simulink model "copper_solvent_extraction_model_simulink"  (R2021a)
settings: Solver=ode14x  StartTime=0.0  StopTime=simulation_time  FixedStep=step_time  RelTol=1e-3
undefined symbols (not defined in the file): C1_aq_ss, C1_el_ss, C1_org_ss, C2_aq_ss, C2_org_ss, C3_aq_ss, C3_org_ss, C4_org_ss, C_aq_max, C_org_max, cLE_ss, cPLS_ss, EXTERNAL_VARIABLES_STEADY_STATE, fLE_max, fLO_max, fPLSP_ss, fPLSS_ss, I_FB1, I_FB2, K_eq_ext, K_eq_str, K_ff_FF1, K_ff_FF2, K_ff_FF3, K_ff_FF4, K_mass_1, K_mass_2, K_mass_3, K_mass_4, Kb_FB1, Kb_FB2, Kc_FB1, Kc_FB2, seed_c_BO, seed_c_LE, seed_c_LO, seed_c_PLS, seed_c_RaffP, seed_c_RaffS, seed_c_RE, seed_f_LE, seed_f_LO, seed_f_PLSP, seed_f_PLSS, sigma_c_BO, sigma_c_LE, sigma_c_LO, sigma_c_PLS, sigma_c_RaffP, sigma_c_RaffS, sigma_c_RE, sigma_f_LE, sigma_f_LO, sigma_f_PLSP, sigma_f_PLSS, step_time, t1, t2, t3, t4 ... (+22)
libraries: slpidlib x2
(part 2 of 2)

== system copper_solvent_extraction_model_simulink/Valve LE ==
  vLE_control_saturated(t) : Inport
  Memory : Memory  InitialCondition=vLE_ss
  Simulation time : Clock
  Valve LE flow model : Subsystem
      mask Display: image('C:\Users\piete\Desktop\Programming\Engineering\Process-State-Identification\assets\simulink\valves\valve_LE_flow_model.png'); % Use "Edit Image" on toolstrip to change.
  Valve LE valve model : Subsystem
      settings: PortSchema="{\"entries\":[{\"content\":{\"sides\":[{\"content\":{\"connectorIds\":[\"In1\"]},\"type\":\"ConnectorPlacement.EquallySpacedRectSide\",\"uuid\":\"2e9f031d-8496-4052-a2e0-829d2345863a\"},{\"content\":{\"connectorIds\":[\"Out1\"],\"side\":\"RIGHT\"},\"type\":\"ConnectorPlacement.EquallySpacedRectSide\",\"uuid\":\"38b5eb17-cc51-4fa3-9394-ca0ed547bb78\"},{\"content\":{\"connectorIds\":[\"In2\",\"In3\"],\"side\":\"TOP\"},\"type\":\"ConnectorPlacement.EquallySpacedRectSide\",\"uuid\":\"bfeaaf73-7bd9-4ee3-b412-f379f1bcce90\"}]},\"type\":\"ConnectorPlacement.EquallySpacedConnector\",\"uuid\":\"a9e57682-026b-43fa-bec2-e5bd18169bdc\"}],\"packageUris\":[\"http://schema.mathworks.com/mf0/Connector/R2020b\"],\"version\":\"1.0\"}"
      mask Display: image('C:\Users\piete\Desktop\Programming\Engineering\Process-State-Identification\assets\simulink\valves\valve_LE_valve_model.png'); % Use "Edit Image" on toolstrip to change.
  Variant Subsystem : Subsystem  Variant=on
      mask Display: image('.\assets\simulink\valves\valve_LE_state.png'); % Use "Edit Image" on toolstrip to change.
  fLE(t) : Outport
  wires:
  Valve LE flow model/1(fLE(t)) -> fLE(t)/1  "fLE(t)"
  Variant Subsystem/1(valve_LE_state) -> Valve LE valve model/2(valve_LE_state)  "valve_LE_state(t)"
  Simulation time/1 -> Variant Subsystem/1(simulation_time)  "simulation_time"
  Variant Subsystem/2(v_LE_is_not_stuck) -> Valve LE valve model/3(v_LE_is_not_stuck(t))  "v_LE_is_not_stuck(t)"
  Memory/1 -> Variant Subsystem/2(v_LE_valve_previous)  "v_LE_valve_previous(t)"
  Valve LE valve model/1(v_LE_valve(t)) -> Memory/1, Valve LE flow model/1(vLE_valve(t))  "v_LE_valve(t)"
  vLE_control_saturated(t)/1 -> Valve LE valve model/1(v_LE_control(t))  "vLE_control_saturated(t)"

== system copper_solvent_extraction_model_simulink/Valve LO ==
  vLO_control_saturated(t) : Inport
  Memory : Memory  InitialCondition=vLO_ss
  Simulation time : Clock
  Valve LO flow model : Subsystem
      mask Display: image('.\assets\simulink\valves\valve_LO_flow_model.png'); % Use "Edit Image" on toolstrip to change.
  Valve LO valve model : Subsystem
      settings: PortSchema="{\"entries\":[{\"content\":{\"sides\":[{\"content\":{\"connectorIds\":[\"In1\"]},\"type\":\"ConnectorPlacement.EquallySpacedRectSide\",\"uuid\":\"2e9f031d-8496-4052-a2e0-829d2345863a\"},{\"content\":{\"connectorIds\":[\"Out1\"],\"side\":\"RIGHT\"},\"type\":\"ConnectorPlacement.EquallySpacedRectSide\",\"uuid\":\"38b5eb17-cc51-4fa3-9394-ca0ed547bb78\"},{\"content\":{\"connectorIds\":[\"In2\",\"In3\"],\"side\":\"TOP\"},\"type\":\"ConnectorPlacement.EquallySpacedRectSide\",\"uuid\":\"bfeaaf73-7bd9-4ee3-b412-f379f1bcce90\"}]},\"type\":\"ConnectorPlacement.EquallySpacedConnector\",\"uuid\":\"a9e57682-026b-43fa-bec2-e5bd18169bdc\"}],\"packageUris\":[\"http://schema.mathworks.com/mf0/Connector/R2020b\"],\"version\":\"1.0\"}"
      mask Display: image('.\assets\simulink\valves\valve_LO_valve_model.png'); % Use "Edit Image" on toolstrip to change.
  Variant Subsystem : Subsystem  Variant=on
      mask Display: image('.\assets\simulink\valves\valve_LO_state.png'); % Use "Edit Image" on toolstrip to change.
  f_LO(t) : Outport
  wires:
  Valve LO flow model/1(fLO(t)) -> f_LO(t)/1  "f_LO(t)"
  vLO_control_saturated(t)/1 -> Valve LO valve model/1(v_LO_control(t))  "vLO_control_saturated(t)"
  Valve LO valve model/1(v_LO_valve(t)) -> Memory/1, Valve LO flow model/1(vLO_valve(t))  "v_LO_valve(t)"
  Variant Subsystem/1(valve_LO_state) -> Valve LO valve model/2(valve_LO_state)  "valve_LO_state(t)"
  Simulation time/1 -> Variant Subsystem/1(simulation_time)  "simulation_time"
  Variant Subsystem/2(v_LO_is_not_stuck) -> Valve LO valve model/3(v_LO_is_not_stuck(t))  "v_LO_is_not_stuck(t)"
  Memory/1 -> Variant Subsystem/2(v_LO_valve_previous)  "v_LO_valve_previous(t)"

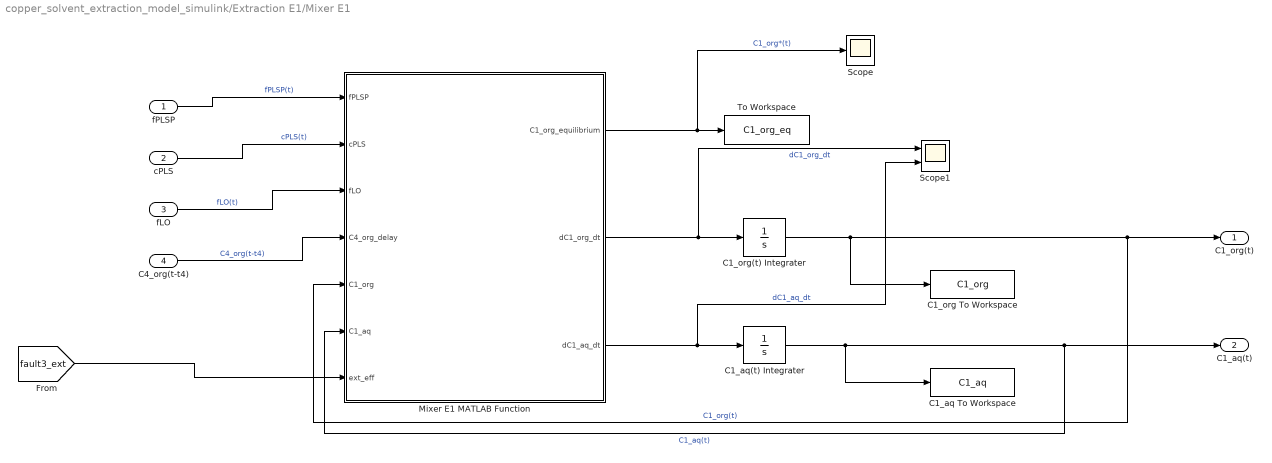
== system copper_solvent_extraction_model_simulink/Extraction E1/Mixer E1 ==
  fPLSP : Inport
  cPLS : Inport  Port=2
  fLO : Inport  Port=3
  C4_org(t-t4) : Inport  Port=4
  C1_aq To Workspace : ToWorkspace  VariableName=C1_aq  SaveFormat=Timeseries  SampleTime=-1
  C1_aq(t) Integrater : Integrator  InitialCondition=C1_aq_ss
  C1_org To Workspace : ToWorkspace  VariableName=C1_org  SaveFormat=Timeseries  SampleTime=-1
  C1_org(t) Integrater : Integrator  InitialCondition=C1_org_ss
  Mixer E1 MATLAB Function : MATLAB Function  TreatAsAtomicUnit=on
  Scope : Scope
  Scope1 : Scope  NumInputPorts=2
  To Workspace : ToWorkspace  VariableName=C1_org_eq  SaveFormat=Timeseries  SampleTime=-1
  C1_org(t) : Outport
  C1_aq(t) : Outport  Port=2
  wires:
  C1_org(t) Integrater/1 -> C1_org(t)/1, Mixer E1 MATLAB Function/5(C1_org), C1_org To Workspace/1  "C1_org(t)"
  Mixer E1 MATLAB Function/2(dC1_org_dt) -> Scope1/1, C1_org(t) Integrater/1  "dC1_org_dt"
  C1_aq(t) Integrater/1 -> C1_aq(t)/1, Mixer E1 MATLAB Function/6(C1_aq), C1_aq To Workspace/1  "C1_aq(t)"
  Mixer E1 MATLAB Function/1(C1_org_equilibrium) -> Scope/1, To Workspace/1  "C1_org*(t)"
  Mixer E1 MATLAB Function/3(dC1_aq_dt) -> Scope1/2, C1_aq(t) Integrater/1  "dC1_aq_dt"
  C4_org(t-t4)/1 -> Mixer E1 MATLAB Function/4(C4_org_delay)  "C4_org(t-t4)"
  fLO/1 -> Mixer E1 MATLAB Function/3(fLO)  "fLO(t)"
  cPLS/1 -> Mixer E1 MATLAB Function/2(cPLS)  "cPLS(t)"
  fPLSP/1 -> Mixer E1 MATLAB Function/1(fPLSP)  "fPLSP(t)"
  [fault3_ext] -> Mixer E1 MATLAB Function/7(ext_eff)

== system copper_solvent_extraction_model_simulink/Extraction E1/Sensor c_RaffP ==
  c_RaffP(t) : Inport
  Random Number : RandomNumber  Variance=sigma_c_RaffP^2  Seed=seed_c_RaffP  SampleTime=step_time
  Saturation : Saturate  UpperLimit=inf  LowerLimit=0
  Sum : Sum  Inputs=++|
  To Workspace : ToWorkspace  VariableName=c_RaffP_measured  SaveFormat=Timeseries  SampleTime=-1
  wires:
  c_RaffP(t)/1 -> Sum/2  "c_RaffP(t)"
  Random Number/1 -> Sum/1  "Sensor c_RaffP Noise"
  Sum/1 -> Saturation/1  "c_RaffP_measured(t)"
  Saturation/1 -> To Workspace/1  "c_RaffP_measured_bounded(t)"

== system copper_solvent_extraction_model_simulink/Extraction E1/Settler E1 ==
  C1_org(t) : Inport
  C1_aq(t) : Inport  Port=2
  C1_aq_delay To Workspace : ToWorkspace  VariableName=C1_aq_delay  SaveFormat=Timeseries  SampleTime=-1
  C1_org_delay To Workspace : ToWorkspace  VariableName=C1_org_delay  SaveFormat=Timeseries  SampleTime=-1
  E1 Aqueous Settler : TransportDelay  DelayTime=t1  InitialOutput=C1_aq_ss
  E1 Organic Settler : TransportDelay  DelayTime=t1  InitialOutput=C1_org_ss
  C1_org(t-t1) : Outport
  C1_aq(t-t1) : Outport  Port=2
  wires:
  C1_org(t)/1 -> E1 Organic Settler/1  "C1_org(t)"
  E1 Organic Settler/1 -> C1_org_delay To Workspace/1, C1_org(t-t1)/1  "C1_org(t-t1)"
  E1 Aqueous Settler/1 -> C1_aq(t-t1)/1, C1_aq_delay To Workspace/1  "C1_aq(t-t1)"
  C1_aq(t)/1 -> E1 Aqueous Settler/1  "C1_aq(t)"

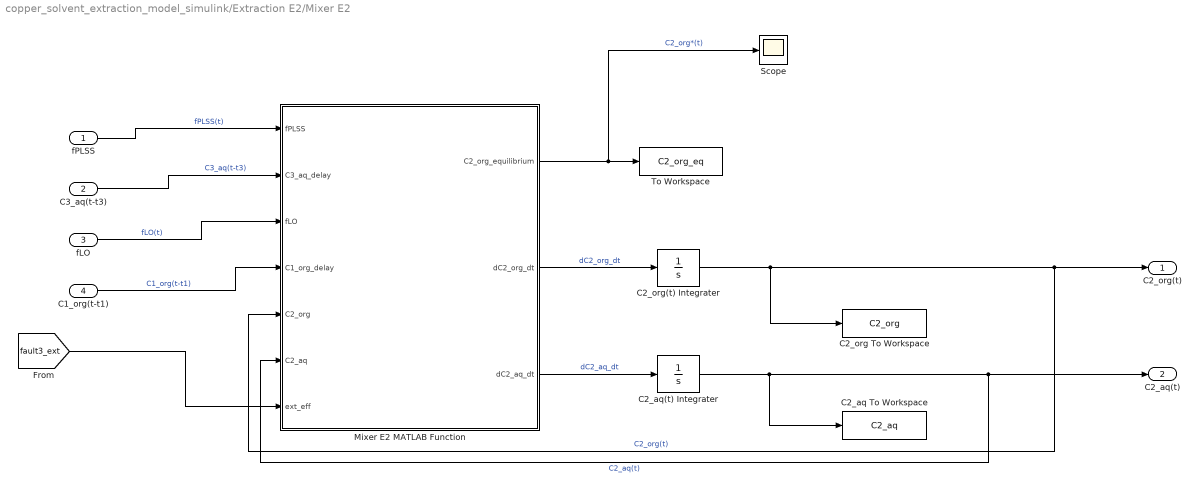
== system copper_solvent_extraction_model_simulink/Extraction E2/Mixer E2 ==
  fPLSS : Inport
  C3_aq(t-t3) : Inport  Port=2
  fLO : Inport  Port=3
  C1_org(t-t1) : Inport  Port=4
  C2_aq To Workspace : ToWorkspace  VariableName=C2_aq  SaveFormat=Timeseries  SampleTime=-1
  C2_aq(t) Integrater : Integrator  InitialCondition=C2_aq_ss
  C2_org To Workspace : ToWorkspace  VariableName=C2_org  SaveFormat=Timeseries  SampleTime=-1
  C2_org(t) Integrater : Integrator  InitialCondition=C2_org_ss
  Mixer E2 MATLAB Function : MATLAB Function  TreatAsAtomicUnit=on
  Scope : Scope
  To Workspace : ToWorkspace  VariableName=C2_org_eq  SaveFormat=Timeseries  SampleTime=-1
  C2_org(t) : Outport
  C2_aq(t) : Outport  Port=2
  wires:
  C2_aq(t) Integrater/1 -> Mixer E2 MATLAB Function/6(C2_aq), C2_aq(t)/1, C2_aq To Workspace/1  "C2_aq(t)"
  C2_org(t) Integrater/1 -> C2_org(t)/1, Mixer E2 MATLAB Function/5(C2_org), C2_org To Workspace/1  "C2_org(t)"
  fLO/1 -> Mixer E2 MATLAB Function/3(fLO)  "fLO(t)"
  Mixer E2 MATLAB Function/3(dC2_aq_dt) -> C2_aq(t) Integrater/1  "dC2_aq_dt"
  Mixer E2 MATLAB Function/1(C2_org_equilibrium) -> Scope/1, To Workspace/1  "C2_org*(t)"
  Mixer E2 MATLAB Function/2(dC2_org_dt) -> C2_org(t) Integrater/1  "dC2_org_dt"
  fPLSS/1 -> Mixer E2 MATLAB Function/1(fPLSS)  "fPLSS(t)"
  C3_aq(t-t3)/1 -> Mixer E2 MATLAB Function/2(C3_aq_delay)  "C3_aq(t-t3)"
  C1_org(t-t1)/1 -> Mixer E2 MATLAB Function/4(C1_org_delay)  "C1_org(t-t1)"
  [fault3_ext] -> Mixer E2 MATLAB Function/7(ext_eff)

== system copper_solvent_extraction_model_simulink/Extraction E2/Sensor c_RaffS ==
  c_RaffS(t) : Inport
  Random Number : RandomNumber  Variance=sigma_c_RaffS^2  Seed=seed_c_RaffS  SampleTime=step_time
  Saturation : Saturate  UpperLimit=inf  LowerLimit=0
  Sum : Sum  Inputs=++|
  To Workspace : ToWorkspace  VariableName=c_RaffS_measured  SaveFormat=Timeseries  SampleTime=-1
  wires:
  c_RaffS(t)/1 -> Sum/2  "c_RaffS(t)"
  Random Number/1 -> Sum/1  "Sensor c_RaffS Noise"
  Sum/1 -> Saturation/1  "c_RaffS_measured(t)"
  Saturation/1 -> To Workspace/1  "c_RaffS_measured_bounded(t)"

== system copper_solvent_extraction_model_simulink/Extraction E2/Settler E2 ==
  C2_org(t) : Inport
  C2_aq(t) : Inport  Port=2
  C2_aq_delay To Workspace : ToWorkspace  VariableName=C2_aq_delay  SaveFormat=Timeseries  SampleTime=-1
  C2_org_delay To Workspace : ToWorkspace  VariableName=C2_org_delay  SaveFormat=Timeseries  SampleTime=-1
  E2 Aqueous Settler : TransportDelay  DelayTime=t2  InitialOutput=C2_aq_ss
  E2 Organic Settler : TransportDelay  DelayTime=t2  InitialOutput=C2_org_ss
  C2_org(t-t2) : Outport
  C2_aq(t-t2) : Outport  Port=2
  wires:
  E2 Aqueous Settler/1 -> C2_aq(t-t2)/1, C2_aq_delay To Workspace/1  "C2_aq(t-t2)"
  C2_aq(t)/1 -> E2 Aqueous Settler/1  "C2_aq(t)"
  C2_org(t)/1 -> E2 Organic Settler/1  "C2_org(t)"
  E2 Organic Settler/1 -> C2_org_delay To Workspace/1, C2_org(t-t2)/1  "C2_org(t-t2)"

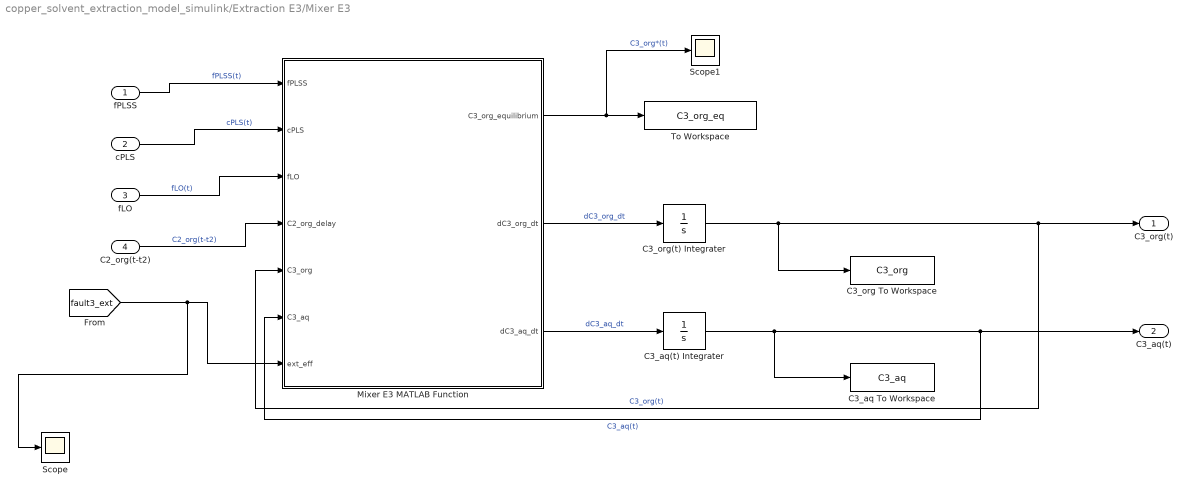
== system copper_solvent_extraction_model_simulink/Extraction E3/Mixer E3 ==
  fPLSS : Inport
  cPLS : Inport  Port=2
  fLO : Inport  Port=3
  C2_org(t-t2) : Inport  Port=4
  C3_aq To Workspace : ToWorkspace  VariableName=C3_aq  SaveFormat=Timeseries  SampleTime=-1
  C3_aq(t) Integrater : Integrator  InitialCondition=C3_aq_ss
  C3_org To Workspace : ToWorkspace  VariableName=C3_org  SaveFormat=Timeseries  SampleTime=-1
  C3_org(t) Integrater : Integrator  InitialCondition=C3_org_ss
  Mixer E3 MATLAB Function : MATLAB Function  TreatAsAtomicUnit=on
  Scope : Scope
  Scope1 : Scope
  To Workspace : ToWorkspace  VariableName=C3_org_eq  SaveFormat=Timeseries  SampleTime=-1
  C3_org(t) : Outport
  C3_aq(t) : Outport  Port=2
  wires:
  C3_aq(t) Integrater/1 -> Mixer E3 MATLAB Function/6(C3_aq), C3_aq(t)/1, C3_aq To Workspace/1  "C3_aq(t)"
  C3_org(t) Integrater/1 -> Mixer E3 MATLAB Function/5(C3_org), C3_org(t)/1, C3_org To Workspace/1  "C3_org(t)"
  Mixer E3 MATLAB Function/2(dC3_org_dt) -> C3_org(t) Integrater/1  "dC3_org_dt"
  C2_org(t-t2)/1 -> Mixer E3 MATLAB Function/4(C2_org_delay)  "C2_org(t-t2)"
  Mixer E3 MATLAB Function/3(dC3_aq_dt) -> C3_aq(t) Integrater/1  "dC3_aq_dt"
  cPLS/1 -> Mixer E3 MATLAB Function/2(cPLS)  "cPLS(t)"
  fLO/1 -> Mixer E3 MATLAB Function/3(fLO)  "fLO(t)"
  fPLSS/1 -> Mixer E3 MATLAB Function/1(fPLSS)  "fPLSS(t)"
  Mixer E3 MATLAB Function/1(C3_org_equilibrium) -> Scope1/1, To Workspace/1  "C3_org*(t)"
  [fault3_ext] -> Scope/1, Mixer E3 MATLAB Function/7(ext_eff)

== system copper_solvent_extraction_model_simulink/Extraction E3/Settler E3 ==
  C3_org(t) : Inport
  C3_aq(t) : Inport  Port=2
  C3_aq_delay To Workspace : ToWorkspace  VariableName=C3_aq_delay  SaveFormat=Timeseries  SampleTime=-1
  C3_org_delay To Workspace : ToWorkspace  VariableName=C3_org_delay  SaveFormat=Timeseries  SampleTime=-1
  E3 Aqueous Settler : TransportDelay  DelayTime=t3  InitialOutput=C3_aq_ss
  E3 Organic Settler : TransportDelay  DelayTime=t3  InitialOutput=C3_org_ss
  C3_org(t-t3) : Outport
  C3_aq(t-t3) : Outport  Port=2
  wires:
  C3_aq(t)/1 -> E3 Aqueous Settler/1  "C3_aq(t)"
  E3 Aqueous Settler/1 -> C3_aq(t-t3)/1, C3_aq_delay To Workspace/1  "C3_aq(t-t3)"
  E3 Organic Settler/1 -> C3_org(t-t3)/1, C3_org_delay To Workspace/1  "C3_org(t-t3)"
  C3_org(t)/1 -> E3 Organic Settler/1  "C3_org(t)"

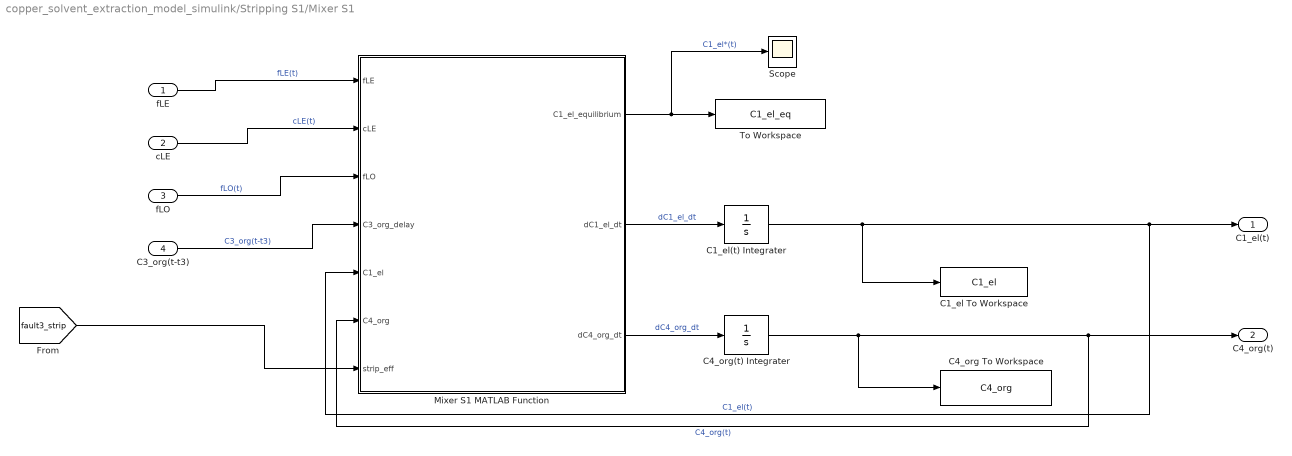
== system copper_solvent_extraction_model_simulink/Stripping S1/Mixer S1 ==
  fLE : Inport
  cLE : Inport  Port=2
  fLO : Inport  Port=3
  C3_org(t-t3) : Inport  Port=4
  C1_el To Workspace : ToWorkspace  VariableName=C1_el  SaveFormat=Timeseries  SampleTime=-1
  C1_el(t) Integrater : Integrator  InitialCondition=C1_el_ss
  C4_org To Workspace : ToWorkspace  VariableName=C4_org  SaveFormat=Timeseries  SampleTime=-1
  C4_org(t) Integrater : Integrator  InitialCondition=C4_org_ss
  Mixer S1 MATLAB Function : MATLAB Function  TreatAsAtomicUnit=on
  Scope : Scope
  To Workspace : ToWorkspace  VariableName=C1_el_eq  SaveFormat=Timeseries  SampleTime=-1
  C1_el(t) : Outport
  C4_org(t) : Outport  Port=2
  wires:
  C3_org(t-t3)/1 -> Mixer S1 MATLAB Function/4(C3_org_delay)  "C3_org(t-t3)"
  Mixer S1 MATLAB Function/2(dC1_el_dt) -> C1_el(t) Integrater/1  "dC1_el_dt"
  C4_org(t) Integrater/1 -> Mixer S1 MATLAB Function/6(C4_org), C4_org(t)/1, C4_org To Workspace/1  "C4_org(t)"
  C1_el(t) Integrater/1 -> Mixer S1 MATLAB Function/5(C1_el), C1_el(t)/1, C1_el To Workspace/1  "C1_el(t)"
  cLE/1 -> Mixer S1 MATLAB Function/2(cLE)  "cLE(t)"
  Mixer S1 MATLAB Function/1(C1_el_equilibrium) -> Scope/1, To Workspace/1  "C1_el*(t)"
  Mixer S1 MATLAB Function/3(dC4_org_dt) -> C4_org(t) Integrater/1  "dC4_org_dt"
  fLO/1 -> Mixer S1 MATLAB Function/3(fLO)  "fLO(t)"
  fLE/1 -> Mixer S1 MATLAB Function/1(fLE)  "fLE(t)"
  [fault3_strip] -> Mixer S1 MATLAB Function/7(strip_eff)

== system copper_solvent_extraction_model_simulink/Stripping S1/Settler S1 ==
  C1_el(t) : Inport
  C4_org(t) : Inport  Port=2
  C1_el_delay To Workspace : ToWorkspace  VariableName=C1_el_delay  SaveFormat=Timeseries  SampleTime=-1
  C4_org_delay To Workspace : ToWorkspace  VariableName=C4_org_delay  SaveFormat=Timeseries  SampleTime=-1
  S1 Electrolyte Settler : TransportDelay  DelayTime=t4  InitialOutput=C1_el_ss
  S1 Organic Settler : TransportDelay  DelayTime=t4  InitialOutput=C4_org_ss
  C1_el(t-t4) : Outport
  C4_org(t-t4) : Outport  Port=2
  wires:
  C4_org(t)/1 -> S1 Organic Settler/1  "C4_org(t)"
  C1_el(t)/1 -> S1 Electrolyte Settler/1  "C1_el(t)"
  S1 Organic Settler/1 -> C4_org(t-t4)/1, C4_org_delay To Workspace/1  "C4_org(t-t4)"
  S1 Electrolyte Settler/1 -> C1_el(t-t4)/1, C1_el_delay To Workspace/1  "C1_el(t-t4)"

== system copper_solvent_extraction_model_simulink/Valve LE/Valve LE flow model ==
  vLE_valve(t) : Inport
  fLE Gain : Gain  Gain=fLE_max
  fLE To Workspace : ToWorkspace  VariableName=fLE  SaveFormat=Timeseries  SampleTime=-1
  fLE(t) : Outport
  wires:
  fLE Gain/1 -> fLE(t)/1, fLE To Workspace/1  "fLE(t)"
  vLE_valve(t)/1 -> fLE Gain/1  "vLE_valve(t)"

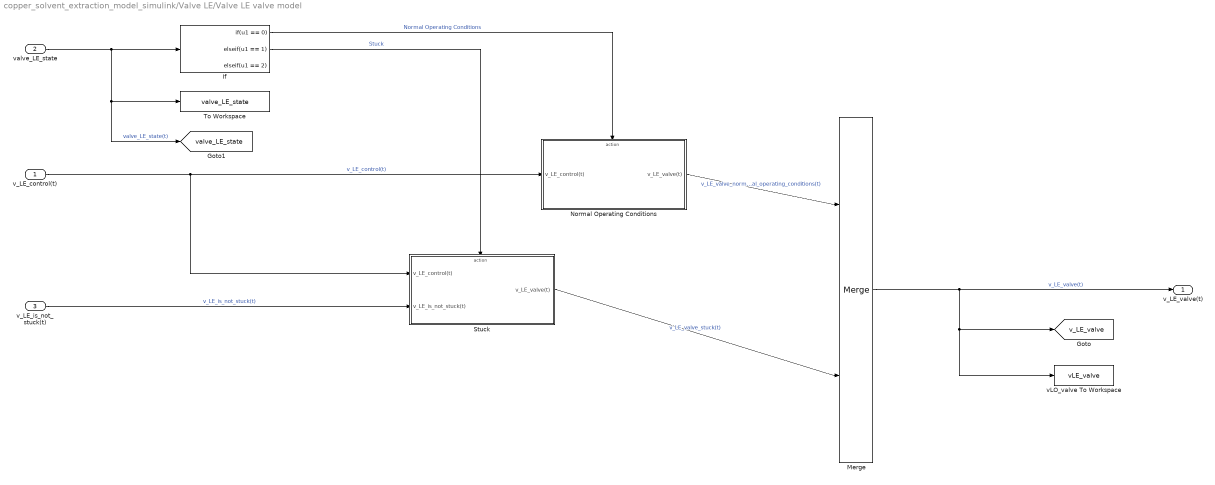
== system copper_solvent_extraction_model_simulink/Valve LE/Valve LE valve model ==
  v_LE_control(t) : Inport
  valve_LE_state : Inport  Port=2
  v_LE_is_not_stuck(t) : Inport  Port=3
  If : If  IfExpression=u1 == 0  ElseIfExpressions=u1 == 1, u1 == 2  ShowElse=off
  Merge : Merge
  Normal Operating Conditions : Subsystem  TreatAsAtomicUnit=on
      mask Display: image('.\assets\simulink\valves\normal.png'); % Use "Edit Image" on toolstrip to change.
  Stuck : Subsystem  TreatAsAtomicUnit=on
      mask Display: image('.\assets\simulink\valves\stuck.png'); % Use "Edit Image" on toolstrip to change.
  To Workspace : ToWorkspace  VariableName=valve_LE_state  SaveFormat=Timeseries  SampleTime=-1
  vLO_valve To Workspace : ToWorkspace  VariableName=vLE_valve  SaveFormat=Timeseries  SampleTime=-1
  v_LE_valve(t) : Outport
  tag scope: v_LE_valve=global, valve_LE_state=global
  wires:
  Merge/1 -> v_LE_valve(t)/1, vLO_valve To Workspace/1, [v_LE_valve]  "v_LE_valve(t)"
  v_LE_control(t)/1 -> Normal Operating Conditions/1(v_LE_control(t)), Stuck/1(v_LE_control(t))  "v_LE_control(t)"
  valve_LE_state/1 -> [valve_LE_state], To Workspace/1, If/1  "valve_LE_state(t)"
  If/1 -> Normal Operating Conditions/Action  "Normal Operating Conditions"
  If/2 -> Stuck/Action  "Stuck"
  Normal Operating Conditions/1(v_LE_valve(t)) -> Merge/1  "v_LE_valve_normal_operating_conditions(t)"
  Stuck/1(v_LE_valve(t)) -> Merge/2  "v_LE_valve_stuck(t)"
  v_LE_is_not_stuck(t)/1 -> Stuck/2(v_LE_is_not_stuck(t))  "v_LE_is_not_stuck(t)"

== system copper_solvent_extraction_model_simulink/Valve LE/Variant Subsystem ==
  simulation_time : Inport
  v_LE_valve_previous : Inport  Port=2
  Valve LE State Custom : Subsystem  VariantControl=VALVE_LE_STATE_CUSTOM
      mask Display: image('.\assets\simulink\valves\custom.png'); % Use "Edit Image" on toolstrip to change.
  Valve LE State Normal : Subsystem  VariantControl=VALVE_LE_STATE_NORMAL
      mask Display: image('.\assets\simulink\valves\normal_variant_subsystem.png'); % Use "Edit Image" on toolstrip to change.
  Valve LE State Stiction : Subsystem  VariantControl=VALVE_LE_STATE_STICTION
      mask Display: image('.\assets\simulink\valves\stiction_variant_subsystem.png'); % Use "Edit Image" on toolstrip to change.
  Valve LE State Stuck : Subsystem  VariantControl=VALVE_LE_STATE_STUCK
      mask Display: image('.\assets\simulink\valves\stuck_variant_subsystem.png'); % Use "Edit Image" on toolstrip to change.
  valve_LE_state : Outport
  v_LE_is_not_stuck : Outport  Port=2
  valve_LE_stiction_v_initial : Outport  Port=3
  valve_LE_stiction_start_time : Outport  Port=4

== system copper_solvent_extraction_model_simulink/Valve LO/Valve LO flow model ==
  vLO_valve(t) : Inport
  fLO Gain : Gain  Gain=fLO_max
  fLO To Workspace : ToWorkspace  VariableName=fLO  SaveFormat=Timeseries  SampleTime=-1
  fLO(t) : Outport
  wires:
  fLO Gain/1 -> fLO(t)/1, fLO To Workspace/1  "fLO(t)"
  vLO_valve(t)/1 -> fLO Gain/1

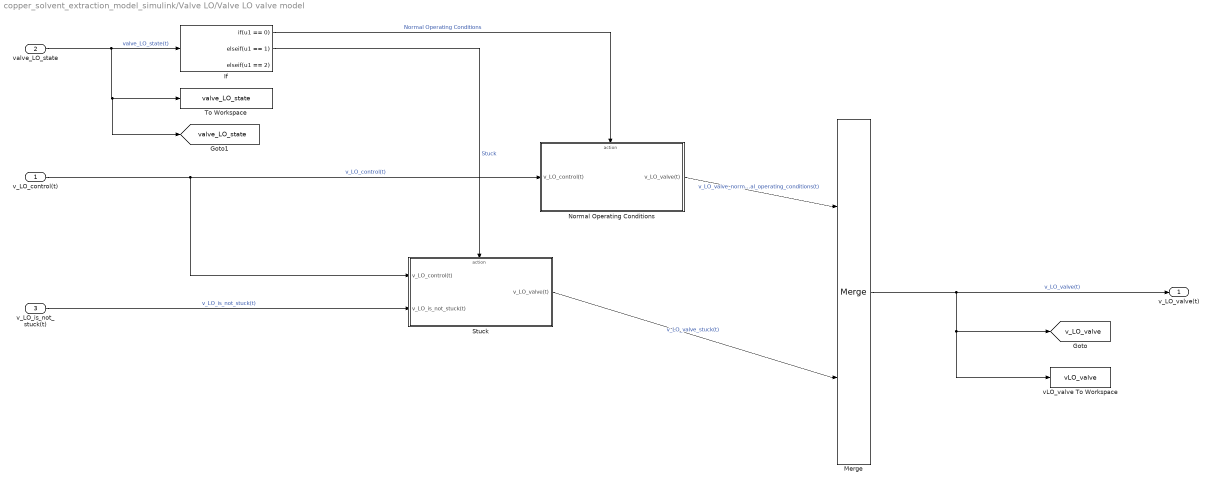
== system copper_solvent_extraction_model_simulink/Valve LO/Valve LO valve model ==
  v_LO_control(t) : Inport
  valve_LO_state : Inport  Port=2
  v_LO_is_not_stuck(t) : Inport  Port=3
  If : If  IfExpression=u1 == 0  ElseIfExpressions=u1 == 1, u1 == 2  ShowElse=off
  Merge : Merge
  Normal Operating Conditions : Subsystem  TreatAsAtomicUnit=on
      mask Display: image('.\assets\simulink\valves\normal.png'); % Use "Edit Image" on toolstrip to change.
  Stuck : Subsystem  TreatAsAtomicUnit=on
      mask Display: image('.\assets\simulink\valves\stuck.png'); % Use "Edit Image" on toolstrip to change.
  To Workspace : ToWorkspace  VariableName=valve_LO_state  SaveFormat=Timeseries  SampleTime=-1
  vLO_valve To Workspace : ToWorkspace  VariableName=vLO_valve  SaveFormat=Timeseries  SampleTime=-1
  v_LO_valve(t) : Outport
  tag scope: v_LO_valve=global, valve_LO_state=global
  wires:
  Merge/1 -> v_LO_valve(t)/1, vLO_valve To Workspace/1, [v_LO_valve]  "v_LO_valve(t)"
  v_LO_control(t)/1 -> Normal Operating Conditions/1(v_LO_control(t)), Stuck/1(v_LO_control(t))  "v_LO_control(t)"
  valve_LO_state/1 -> [valve_LO_state], To Workspace/1, If/1  "valve_LO_state(t)"
  If/1 -> Normal Operating Conditions/Action  "Normal Operating Conditions"
  If/2 -> Stuck/Action  "Stuck"
  Normal Operating Conditions/1(v_LO_valve(t)) -> Merge/1  "v_LO_valve_normal_operating_conditions(t)"
  Stuck/1(v_LO_valve(t)) -> Merge/2  "v_LO_valve_stuck(t)"
  v_LO_is_not_stuck(t)/1 -> Stuck/2(v_LO_is_not_stuck(t))  "v_LO_is_not_stuck(t)"

== system copper_solvent_extraction_model_simulink/Valve LO/Variant Subsystem ==
  simulation_time : Inport
  v_LO_valve_previous : Inport  Port=2
  Valve LO State Custom : Subsystem  VariantControl=VALVE_LO_STATE_CUSTOM
      mask Display: image('.\assets\simulink\valves\custom.png'); % Use "Edit Image" on toolstrip to change.
  Valve LO State Normal : Subsystem  VariantControl=VALVE_LO_STATE_NORMAL
      mask Display: image('.\assets\simulink\valves\normal_variant_subsystem.png'); % Use "Edit Image" on toolstrip to change.
  Valve LO State Stiction : Subsystem  VariantControl=VALVE_LO_STATE_STICTION
      mask Display: image('.\assets\simulink\valves\stiction_variant_subsystem.png'); % Use "Edit Image" on toolstrip to change.
  Valve LO State Stuck : Subsystem  VariantControl=VALVE_LO_STATE_STUCK
      mask Display: image('.\assets\simulink\valves\stuck_variant_subsystem.png'); % Use "Edit Image" on toolstrip to change.
  valve_LO_state : Outport
  v_LO_is_not_stuck : Outport  Port=2
  valve_LO_stiction_v_initial : Outport  Port=3
  valve_LO_stiction_start_time : Outport  Port=4

== system copper_solvent_extraction_model_simulink/Valve LE/Valve LE valve model/Normal Operating Conditions ==
  v_LE_control(t) : Inport
  Action Port : ActionPort  ActionPortLabel=if(u1 == 0)
  LE Valve Model : Gain
  v_LE_valve(t) : Outport
  wires:
  LE Valve Model/1 -> v_LE_valve(t)/1  "v_LE_valve(t)"
  v_LE_control(t)/1 -> LE Valve Model/1  "v_LE_control(t)"

== system copper_solvent_extraction_model_simulink/Valve LE/Valve LE valve model/Stuck ==
  v_LE_control(t) : Inport
  v_LE_is_not_stuck(t) : Inport  Port=2
  Action Port : ActionPort  ActionPortLabel=elseif(u1 == 1)
  Memory : Memory  InitialCondition=vLE_ss
  Switch : Switch  Criteria=u2 > Threshold
  v_LE_valve(t) : Outport
  wires:
  v_LE_control(t)/1 -> Switch/1  "v_LE_control(t)"
  Switch/1 -> v_LE_valve(t)/1, Memory/1  "v_LE_valve(t)"
  Memory/1 -> Switch/3  "v_LE_valve_previous(t)"
  v_LE_is_not_stuck(t)/1 -> Switch/2  "v_LE_is_not_stuck(t)"

== system copper_solvent_extraction_model_simulink/Valve LE/Variant Subsystem/Valve LE State Custom ==
  simulation_time : Inport
  v_LE_valve_previous : Inport  Port=2
  Valve LE Finite State Machine Custom : Stateflow chart  TreatAsAtomicUnit=on
  valve_LE_state : Outport
  v_LE_is_not_stuck : Outport  Port=2
  valve_LE_stiction_v_initial : Outport  Port=3
  valve_LE_stiction_start_time : Outport  Port=4
  wires:
  Valve LE Finite State Machine Custom/1(valve_LE_state) -> valve_LE_state/1  "valve_LE_state(t)"
  Valve LE Finite State Machine Custom/2(v_LE_is_not_stuck) -> v_LE_is_not_stuck/1  "v_LE_is_not_stuck(t)"
  Valve LE Finite State Machine Custom/3(valve_LE_stiction_v_initial) -> valve_LE_stiction_v_initial/1  "valve_LE_stiction_v_initial"
  Valve LE Finite State Machine Custom/4(valve_LE_stiction_start_time) -> valve_LE_stiction_start_time/1  "valve_LE_stiction_start_time"
  v_LE_valve_previous/1 -> Valve LE Finite State Machine Custom/2(v_LE_valve_previous)  "v_LE_valve_previous"
  simulation_time/1 -> Valve LE Finite State Machine Custom/1(simulation_time)  "simulation_time"

== system copper_solvent_extraction_model_simulink/Valve LE/Variant Subsystem/Valve LE State Normal ==
  simulation_time : Inport
  v_LE_valve_previous : Inport  Port=2
  Valve LE Finite State Machine Normal : Stateflow chart  TreatAsAtomicUnit=on
  valve_LE_state : Outport
  v_LE_is_not_stuck : Outport  Port=2
  valve_LE_stiction_v_initial : Outport  Port=3
  valve_LE_stiction_start_time : Outport  Port=4
  wires:
  Valve LE Finite State Machine Normal/1(valve_LE_state) -> valve_LE_state/1  "valve_LE_state(t)"
  Valve LE Finite State Machine Normal/2(v_LE_is_not_stuck) -> v_LE_is_not_stuck/1  "v_LE_is_not_stuck(t)"
  Valve LE Finite State Machine Normal/3(valve_LE_stiction_v_initial) -> valve_LE_stiction_v_initial/1  "valve_LE_stiction_v_initial"
  Valve LE Finite State Machine Normal/4(valve_LE_stiction_start_time) -> valve_LE_stiction_start_time/1  "valve_LE_stiction_start_time"
  v_LE_valve_previous/1 -> Valve LE Finite State Machine Normal/2(v_LE_valve_previous)  "v_LE_valve_previous"
  simulation_time/1 -> Valve LE Finite State Machine Normal/1(simulation_time)  "simulation_time"

== system copper_solvent_extraction_model_simulink/Valve LE/Variant Subsystem/Valve LE State Stiction ==
  simulation_time : Inport
  v_LE_valve_previous : Inport  Port=2
  Valve LE Finite State Machine Stiction : Stateflow chart  TreatAsAtomicUnit=on
  valve_LE_state : Outport
  v_LE_is_not_stuck : Outport  Port=2
  valve_LE_stiction_v_initial : Outport  Port=3
  valve_LE_stiction_start_time : Outport  Port=4
  wires:
  Valve LE Finite State Machine Stiction/1(valve_LE_state) -> valve_LE_state/1  "valve_LE_state(t)"
  Valve LE Finite State Machine Stiction/2(v_LE_is_not_stuck) -> v_LE_is_not_stuck/1  "v_LE_is_not_stuck(t)"
  Valve LE Finite State Machine Stiction/3(valve_LE_stiction_v_initial) -> valve_LE_stiction_v_initial/1  "valve_LE_stiction_v_initial"
  Valve LE Finite State Machine Stiction/4(valve_LE_stiction_start_time) -> valve_LE_stiction_start_time/1  "valve_LE_stiction_start_time"
  v_LE_valve_previous/1 -> Valve LE Finite State Machine Stiction/2(v_LE_valve_previous)  "v_LE_valve_previous"
  simulation_time/1 -> Valve LE Finite State Machine Stiction/1(simulation_time)  "simulation_time"

== system copper_solvent_extraction_model_simulink/Valve LE/Variant Subsystem/Valve LE State Stuck ==
  simulation_time : Inport
  v_LE_valve_previous : Inport  Port=2
  Valve LE Finite State Machine Stuck : Stateflow chart  TreatAsAtomicUnit=on
  valve_LE_state : Outport
  v_LE_is_not_stuck : Outport  Port=2
  valve_LE_stiction_v_initial : Outport  Port=3
  valve_LE_stiction_start_time : Outport  Port=4
  wires:
  Valve LE Finite State Machine Stuck/1(valve_LE_state) -> valve_LE_state/1  "valve_LE_state(t)"
  Valve LE Finite State Machine Stuck/2(v_LE_is_not_stuck) -> v_LE_is_not_stuck/1  "v_LE_is_not_stuck(t)"
  Valve LE Finite State Machine Stuck/3(valve_LE_stiction_v_initial) -> valve_LE_stiction_v_initial/1  "valve_LE_stiction_v_initial"
  Valve LE Finite State Machine Stuck/4(valve_LE_stiction_start_time) -> valve_LE_stiction_start_time/1  "valve_LE_stiction_start_time"
  v_LE_valve_previous/1 -> Valve LE Finite State Machine Stuck/2(v_LE_valve_previous)  "v_LE_valve_previous"
  simulation_time/1 -> Valve LE Finite State Machine Stuck/1(simulation_time)  "simulation_time"

== system copper_solvent_extraction_model_simulink/Valve LO/Valve LO valve model/Normal Operating Conditions ==
  v_LO_control(t) : Inport
  Action Port : ActionPort  ActionPortLabel=if(u1 == 0)
  LO Valve Model : Gain
  v_LO_valve(t) : Outport
  wires:
  LO Valve Model/1 -> v_LO_valve(t)/1  "v_LO_valve(t)"
  v_LO_control(t)/1 -> LO Valve Model/1  "v_LO_control(t)"

== system copper_solvent_extraction_model_simulink/Valve LO/Valve LO valve model/Stuck ==
  v_LO_control(t) : Inport
  v_LO_is_not_stuck(t) : Inport  Port=2
  Action Port : ActionPort  ActionPortLabel=elseif(u1 == 1)
  Memory : Memory  InitialCondition=vLO_ss
  Switch : Switch  Criteria=u2 > Threshold
  v_LO_valve(t) : Outport
  wires:
  v_LO_control(t)/1 -> Switch/1  "v_LO_control(t)"
  Switch/1 -> v_LO_valve(t)/1, Memory/1  "v_LO_valve(t)"
  Memory/1 -> Switch/3  "v_LO_valve_previous(t)"
  v_LO_is_not_stuck(t)/1 -> Switch/2  "v_LO_is_not_stuck(t)"

== system copper_solvent_extraction_model_simulink/Valve LO/Variant Subsystem/Valve LO State Custom ==
  simulation_time : Inport
  v_LO_valve_previous : Inport  Port=2
  Valve LO Finite State Machine Custom : Stateflow chart  TreatAsAtomicUnit=on
  valve_LO_state : Outport
  v_LO_is_not_stuck : Outport  Port=2
  valve_LO_stiction_v_initial : Outport  Port=3
  valve_LO_stiction_start_time : Outport  Port=4
  wires:
  Valve LO Finite State Machine Custom/1(valve_LO_state) -> valve_LO_state/1  "valve_LO_state(t)"
  Valve LO Finite State Machine Custom/2(v_LO_is_not_stuck) -> v_LO_is_not_stuck/1  "v_LO_is_not_stuck(t)"
  Valve LO Finite State Machine Custom/3(valve_LO_stiction_v_initial) -> valve_LO_stiction_v_initial/1  "valve_LO_stiction_v_initial"
  Valve LO Finite State Machine Custom/4(valve_LO_stiction_start_time) -> valve_LO_stiction_start_time/1  "valve_LO_stiction_start_time"
  v_LO_valve_previous/1 -> Valve LO Finite State Machine Custom/2(v_LO_valve_previous)  "v_LO_valve_previous"
  simulation_time/1 -> Valve LO Finite State Machine Custom/1(simulation_time)  "simulation_time"

== system copper_solvent_extraction_model_simulink/Valve LO/Variant Subsystem/Valve LO State Normal ==
  simulation_time : Inport
  v_LO_valve_previous : Inport  Port=2
  Valve LO Finite State Machine Normal : Stateflow chart  TreatAsAtomicUnit=on
  valve_LO_state : Outport
  v_LO_is_not_stuck : Outport  Port=2
  valve_LO_stiction_v_initial : Outport  Port=3
  valve_LO_stiction_start_time : Outport  Port=4
  wires:
  Valve LO Finite State Machine Normal/1(valve_LO_state) -> valve_LO_state/1  "valve_LO_state(t)"
  Valve LO Finite State Machine Normal/2(v_LO_is_not_stuck) -> v_LO_is_not_stuck/1  "v_LO_is_not_stuck(t)"
  Valve LO Finite State Machine Normal/3(valve_LO_stiction_v_initial) -> valve_LO_stiction_v_initial/1  "valve_LO_stiction_v_initial"
  Valve LO Finite State Machine Normal/4(valve_LO_stiction_start_time) -> valve_LO_stiction_start_time/1  "valve_LO_stiction_start_time"
  v_LO_valve_previous/1 -> Valve LO Finite State Machine Normal/2(v_LO_valve_previous)  "v_LO_valve_previous"
  simulation_time/1 -> Valve LO Finite State Machine Normal/1(simulation_time)  "simulation_time"

== system copper_solvent_extraction_model_simulink/Valve LO/Variant Subsystem/Valve LO State Stiction ==
  simulation_time : Inport
  v_LO_valve_previous : Inport  Port=2
  Valve LO Finite State Machine Stiction : Stateflow chart  TreatAsAtomicUnit=on
  valve_LO_state : Outport
  v_LO_is_not_stuck : Outport  Port=2
  valve_LO_stiction_v_initial : Outport  Port=3
  valve_LO_stiction_start_time : Outport  Port=4
  wires:
  Valve LO Finite State Machine Stiction/1(valve_LO_state) -> valve_LO_state/1  "valve_LO_state(t)"
  Valve LO Finite State Machine Stiction/2(v_LO_is_not_stuck) -> v_LO_is_not_stuck/1  "v_LO_is_not_stuck(t)"
  Valve LO Finite State Machine Stiction/3(valve_LO_stiction_v_initial) -> valve_LO_stiction_v_initial/1  "valve_LO_stiction_v_initial"
  Valve LO Finite State Machine Stiction/4(valve_LO_stiction_start_time) -> valve_LO_stiction_start_time/1  "valve_LO_stiction_start_time"
  v_LO_valve_previous/1 -> Valve LO Finite State Machine Stiction/2(v_LO_valve_previous)  "v_LO_valve_previous"
  simulation_time/1 -> Valve LO Finite State Machine Stiction/1(simulation_time)  "simulation_time"

== system copper_solvent_extraction_model_simulink/Valve LO/Variant Subsystem/Valve LO State Stuck ==
  simulation_time : Inport
  v_LO_valve_previous : Inport  Port=2
  Valve LO Finite State Machine Stuck : Stateflow chart  TreatAsAtomicUnit=on
  valve_LO_state : Outport
  v_LO_is_not_stuck : Outport  Port=2
  valve_LO_stiction_v_initial : Outport  Port=3
  valve_LO_stiction_start_time : Outport  Port=4
  wires:
  Valve LO Finite State Machine Stuck/1(valve_LO_state) -> valve_LO_state/1  "valve_LO_state(t)"
  Valve LO Finite State Machine Stuck/2(v_LO_is_not_stuck) -> v_LO_is_not_stuck/1  "v_LO_is_not_stuck(t)"
  Valve LO Finite State Machine Stuck/3(valve_LO_stiction_v_initial) -> valve_LO_stiction_v_initial/1  "valve_LO_stiction_v_initial"
  Valve LO Finite State Machine Stuck/4(valve_LO_stiction_start_time) -> valve_LO_stiction_start_time/1  "valve_LO_stiction_start_time"
  v_LO_valve_previous/1 -> Valve LO Finite State Machine Stuck/2(v_LO_valve_previous)  "v_LO_valve_previous"
  simulation_time/1 -> Valve LO Finite State Machine Stuck/1(simulation_time)  "simulation_time"

== matlab function copper_solvent_extraction_model_simulink/Stripping S1/Mixer S1/Mixer S1 MATLAB Function ==
  data: fLE input; cLE input; fLO input; C3_org_delay input; C1_el input; C4_org input; C1_el_equilibrium output; K_mass_4 parameter; V4 parameter; dC1_el_dt output; dC4_org_dt output; C_aq_max parameter; K_eq_str parameter; strip_eff input
function [C1_el_equilibrium, dC1_el_dt, dC4_org_dt] = fcn(fLE, cLE, fLO, C3_org_delay, C1_el, C4_org, K_mass_4, V4, C_aq_max, K_eq_str, strip_eff)

% Stripping unit S1's Mixer

% The parameters are imported from the workspace, therefore run the
% simulation from the /process_model/copper_solvent_extraction_model.mlx
% live script.

% Dynamic equilibrium
C1_el_equilibrium  = ((C_aq_max * C4_org)./((1./K_eq_str) + C4_org))*strip_eff;

% Mass balances 
dC1_el_dt  = (fLE/V4)*(cLE - C1_el)           + K_mass_4*(C1_el_equilibrium - C1_el);
dC4_org_dt = (fLO/V4)*(C3_org_delay - C4_org) - K_mass_4*(C1_el_equilibrium - C1_el);

end

== matlab function copper_solvent_extraction_model_simulink/Extraction E1/Mixer E1/Mixer E1 MATLAB Function ==
  data: fPLSP input; cPLS input; C1_org_equilibrium output; fLO input; C4_org_delay input; C1_org input; C1_aq input; dC1_org_dt output; K_mass_1 parameter; V1 parameter; dC1_aq_dt output; C_org_max parameter; K_eq_ext parameter; ext_eff input
function [C1_org_equilibrium, dC1_org_dt, dC1_aq_dt] = fcn(fPLSP, cPLS, fLO, C4_org_delay, C1_org, C1_aq, K_mass_1, V1, C_org_max, K_eq_ext, ext_eff)

% Extraction unit E1's Mixer

% The parameters are imported from the workspace, therefore run the
% simulation from the /process_model/copper_solvent_extraction_model.mlx
% live script.

% Dynamic equilibrium
C1_org_equilibrium = ((C_org_max * C1_aq)./((1./(K_eq_ext*ext_eff)) + C1_aq));

% Mass balances 
dC1_org_dt = (fLO/V1)*(C4_org_delay - C1_org) + K_mass_1*(C1_org_equilibrium - C1_org);
dC1_aq_dt  = (fPLSP/V1)*(cPLS - C1_aq)        - K_mass_1*(C1_org_equilibrium - C1_org);

end

== matlab function copper_solvent_extraction_model_simulink/Faults/MATLAB Function ==
  data: fault1_state output; fault2_state output; fault3_ext_state output; fault1 input; fault2 input; fault3_ext input; fault3_strip_state output; fault3_strip input
function [fault1_state, fault2_state, fault3_ext_state, fault3_strip_state]= fcn(fault1, fault2, fault3_ext, fault3_strip)
    if fault1 > 1
        fault1_state = 1;
    else 
        fault1_state = 0;
    end 
    if fault2 > 1
        fault2_state = 1;
    else 
        fault2_state = 0;
    end 
    fault3_ext_state = fault3_ext;
    fault3_strip_state = fault3_strip;

== stateflow chart copper_solvent_extraction_model_simulink/Valve LO/Variant Subsystem/Valve LO State Stuck/Valve LO Finite State Machine Stuck ==
  state Normal
    entry, during:
    valve_LO_state = 0;
    v_LO_is_not_stuck = 1;
  state Stuck
    entry:
    valve_LO_state = 1;
    during:
    valve_LO_state = 1;
    v_LO_is_not_stuck = 0;
  state Stiction
    entry:
    valve_LO_state = 2;
    valve_LO_stiction_v_initial = v_LO_valve_previous;
    valve_LO_stiction_start_time = simulation_time;
    during:
    valve_LO_state = 2;
  (default) -> Normal
  Normal -> Stuck : [simulation_time == valve_LO_fault_start_time]
  Stuck -> Normal : [simulation_time == valve_LO_fault_stop_time]
  data: valve_LO_state output; simulation_time input; v_LO_is_not_stuck output; valve_LO_fault_start_time parameter; valve_LO_fault_stop_time parameter; valve_LO_stiction_v_initial output; v_LO_valve_previous input; valve_LO_stiction_start_time output

== stateflow chart copper_solvent_extraction_model_simulink/Valve LO/Variant Subsystem/Valve LO State Stiction/Valve LO Finite State Machine Stiction ==
  state Normal
    entry, during:
    valve_LO_state = 0;
    v_LO_is_not_stuck = 1;
  state Stuck
    entry:
    valve_LO_state = 1;
    during:
    valve_LO_state = 1;
    v_LO_is_not_stuck = 0;
  state Stiction
    entry:
    valve_LO_state = 2;
    valve_LO_stiction_v_initial = v_LO_valve_previous;
    valve_LO_stiction_start_time = simulation_time;
    during:
    valve_LO_state = 2;
  (default) -> Normal
  Normal -> Stiction : [simulation_time == valve_LO_fault_start_time]
  Stiction -> Normal : [simulation_time == valve_LO_fault_stop_time]
  data: valve_LO_state output; simulation_time input; v_LO_is_not_stuck output; valve_LO_fault_start_time parameter; valve_LO_fault_stop_time parameter; valve_LO_stiction_v_initial output; v_LO_valve_previous input; valve_LO_stiction_start_time output

== stateflow chart copper_solvent_extraction_model_simulink/Valve LE/Variant Subsystem/Valve LE State Normal/Valve LE Finite State Machine Normal ==
  state Normal
    entry, during:
    valve_LE_state = 0;
    v_LE_is_not_stuck = 1;
  state Stuck
    entry:
    valve_LE_state = 1;
    during:
    valve_LE_state = 1;
    v_LE_is_not_stuck = 0;
  state Stiction
    entry:
    valve_LE_state = 2;
    valve_LE_stiction_v_initial = v_LE_valve_previous;
    valve_LE_stiction_start_time = simulation_time;
    during:
    valve_LE_state = 2;
  (default) -> Normal
  data: valve_LE_state output; simulation_time input; v_LE_is_not_stuck output; valve_LE_fault_start_time parameter; valve_LE_fault_stop_time parameter; valve_LE_stiction_v_initial output; v_LE_valve_previous input; valve_LE_stiction_start_time output

== stateflow chart copper_solvent_extraction_model_simulink/Valve LE/Variant Subsystem/Valve LE State Stiction/Valve LE Finite State Machine Stiction ==
  state Normal
    entry, during:
    valve_LE_state = 0;
    v_LE_is_not_stuck = 1;
  state Stuck
    entry:
    valve_LE_state = 1;
    during:
    valve_LE_state = 1;
    v_LE_is_not_stuck = 0;
  state Stiction
    entry:
    valve_LE_state = 2;
    valve_LE_stiction_v_initial = v_LE_valve_previous;
    valve_LE_stiction_start_time = simulation_time;
    during:
    valve_LE_state = 2;
  (default) -> Normal
  Normal -> Stiction : [simulation_time == valve_LE_fault_start_time]
  Stiction -> Normal : [simulation_time == valve_LE_fault_stop_time]
  data: valve_LE_state output; simulation_time input; v_LE_is_not_stuck output; valve_LE_fault_start_time parameter; valve_LE_fault_stop_time parameter; valve_LE_stiction_v_initial output; v_LE_valve_previous input; valve_LE_stiction_start_time output

== stateflow chart copper_solvent_extraction_model_simulink/Valve LE/Variant Subsystem/Valve LE State Stuck/Valve LE Finite State Machine Stuck ==
  state Normal
    entry, during:
    valve_LE_state = 0;
    v_LE_is_not_stuck = 1;
  state Stuck
    entry:
    valve_LE_state = 1;
    during:
    valve_LE_state = 1;
    v_LE_is_not_stuck = 0;
  state Stiction
    entry:
    valve_LE_state = 2;
    valve_LE_stiction_v_initial = v_LE_valve_previous;
    valve_LE_stiction_start_time = simulation_time;
    during:
    valve_LE_state = 2;
  (default) -> Normal
  Normal -> Stuck : [simulation_time == valve_LE_fault_start_time]
  Stuck -> Normal : [simulation_time == valve_LE_fault_stop_time]
  data: valve_LE_state output; simulation_time input; v_LE_is_not_stuck output; valve_LE_fault_start_time parameter; valve_LE_fault_stop_time parameter; valve_LE_stiction_v_initial output; v_LE_valve_previous input; valve_LE_stiction_start_time output

== matlab function copper_solvent_extraction_model_simulink/Simulation Scopes/MATLAB Function ==
  data: valve_LO_state input; simulation_process_state output; valve_LE_state input
function simulation_process_state = fcn(valve_LO_state, valve_LE_state)

    % Initial value
    simulation_process_state = 0;    

    % Process state 0
    if((valve_LO_state == 0) && (valve_LE_state == 0))
        simulation_process_state = 0;
    end
    
    % Process state 1
    if((valve_LO_state == 1) && (valve_LE_state == 0))
        simulation_process_state = 1;
    end
    
    % Process state 2
    if((valve_LO_state == 2) && (valve_LE_state == 0))
        simulation_process_state = 2;
    end
    
    % Process state 3
    if((valve_LO_state == 0) && (valve_LE_state == 1))
        simulation_process_state = 3;
    end
    
    % Process state 4
    if((valve_LO_state == 0) && (valve_LE_state == 2))
        simulation_process_state = 4;
    end
    
    % Process state 5
    if((valve_LO_state == 1) && (valve_LE_state == 1))
        simulation_process_state = 5;
    end
    
    % Process state 6
    if((valve_LO_state == 1) && (valve_LE_state == 2))
        simulation_process_state = 6;
    end
    
    % Process state 7
    if((valve_LO_state == 2) && (valve_LE_state == 1))
        simulation_process_state = 7;
    end
    
    % Process state 8
    if((valve_LO_state == 2) && (valve_LE_state == 2))
        simulation_process_state = 8;
    end
    
end

== stateflow chart copper_solvent_extraction_model_simulink/Valve LO/Variant Subsystem/Valve LO State Custom/Valve LO Finite State Machine Custom ==
  state Normal
    entry, during:
    valve_LO_state = 0;
    v_LO_is_not_stuck = 1;
  state Stuck
    entry:
    valve_LO_state = 1;
    during:
    valve_LO_state = 1;
    v_LO_is_not_stuck = 0;
  state Stiction
    entry:
    valve_LO_state = 2;
    valve_LO_stiction_v_initial = v_LO_valve_previous;
    valve_LO_stiction_start_time = simulation_time;
    during:
    valve_LO_state = 2;
  (default) -> Normal
  Normal -> Stiction : [simulation_time == valve_LO_fault_start_time]
  Stiction -> Normal : [simulation_time == valve_LO_fault_stop_time]
  data: valve_LO_state output; simulation_time input; v_LO_is_not_stuck output; valve_LO_fault_start_time parameter; valve_LO_fault_stop_time parameter; valve_LO_stiction_v_initial output; v_LO_valve_previous input; valve_LO_stiction_start_time output

== stateflow chart copper_solvent_extraction_model_simulink/Valve LE/Variant Subsystem/Valve LE State Custom/Valve LE Finite State Machine Custom ==
  state Normal
    entry, during:
    valve_LE_state = 0;
    v_LE_is_not_stuck = 1;
  state Stuck
    entry:
    valve_LE_state = 1;
    during:
    valve_LE_state = 1;
    v_LE_is_not_stuck = 0;
  state Stiction
    entry:
    valve_LE_state = 2;
    valve_LE_stiction_v_initial = v_LE_valve_previous;
    valve_LE_stiction_start_time = simulation_time;
    during:
    valve_LE_state = 2;
  (default) -> Normal
  Normal -> Stiction : [simulation_time == valve_LE_fault_start_time]
  Stiction -> Normal : [simulation_time == valve_LE_fault_stop_time]
  data: valve_LE_state output; simulation_time input; v_LE_is_not_stuck output; valve_LE_fault_start_time parameter; valve_LE_fault_stop_time parameter; valve_LE_stiction_v_initial output; v_LE_valve_previous input; valve_LE_stiction_start_time output

== matlab function copper_solvent_extraction_model_simulink/Extraction E2/Mixer E2/Mixer E2 MATLAB Function ==
  data: fPLSS input; C3_aq_delay input; fLO input; C1_org_delay input; C2_org input; C2_org_equilibrium output; C2_aq input; K_mass_2 parameter; V2 parameter; dC2_org_dt output; dC2_aq_dt output; C_org_max parameter; K_eq_ext parameter; ext_eff input
function [C2_org_equilibrium, dC2_org_dt, dC2_aq_dt] = fcn(fPLSS, C3_aq_delay, fLO, C1_org_delay, C2_org, C2_aq, K_mass_2, V2, C_org_max, K_eq_ext, ext_eff)

% Extraction unit E2's Mixer

% The parameters are imported from the workspace, therefore run the
% simulation from the /process_model/copper_solvent_extraction_model.mlx
% live script.

% Dynamic equilibrium
C2_org_equilibrium = ((C_org_max * C2_aq)./(1./((K_eq_ext*ext_eff)) + C2_aq));

% Mass balances 
dC2_org_dt = (fLO/V2)*(C1_org_delay - C2_org) + K_mass_2*(C2_org_equilibrium - C2_org);
dC2_aq_dt  = (fPLSS/V2)*(C3_aq_delay - C2_aq) - K_mass_2*(C2_org_equilibrium - C2_org);

end

== stateflow chart copper_solvent_extraction_model_simulink/Valve LO/Variant Subsystem/Valve LO State Normal/Valve LO Finite State Machine Normal ==
  state Normal
    entry, during:
    valve_LO_state = 0;
    v_LO_is_not_stuck = 1;
  state Stuck
    entry:
    valve_LO_state = 1;
    during:
    valve_LO_state = 1;
    v_LO_is_not_stuck = 0;
  state Stiction
    entry:
    valve_LO_state = 2;
    valve_LO_stiction_v_initial = v_LO_valve_previous;
    valve_LO_stiction_start_time = simulation_time;
    during:
    valve_LO_state = 2;
  (default) -> Normal
  data: valve_LO_state output; simulation_time input; v_LO_is_not_stuck output; valve_LO_fault_start_time parameter; valve_LO_fault_stop_time parameter; valve_LO_stiction_v_initial output; v_LO_valve_previous input; valve_LO_stiction_start_time output

== matlab function copper_solvent_extraction_model_simulink/Extraction E3/Mixer E3/Mixer E3 MATLAB Function ==
  data: fPLSS input; cPLS input; C3_org_equilibrium output; fLO input; C2_org_delay input; C3_org input; C3_aq input; K_mass_3 parameter; V3 parameter; dC3_org_dt output; dC3_aq_dt output; C_org_max parameter; K_eq_ext parameter; ext_eff input
function [C3_org_equilibrium, dC3_org_dt, dC3_aq_dt] = fcn(fPLSS, cPLS, fLO, C2_org_delay, C3_org, C3_aq, K_mass_3, V3, C_org_max, K_eq_ext, ext_eff)

% Extraction unit E3's Mixer

% The parameters are imported from the workspace, therefore run the
% simulation from the /process_model/copper_solvent_extraction_model.mlx
% live script.

% Dynamic equilibrium
C3_org_equilibrium = ((C_org_max * C3_aq)./((1./K_eq_ext) + C3_aq))*ext_eff;

% Mass balances 
dC3_org_dt = (fLO/V3)*(C2_org_delay - C3_org) + K_mass_3*(C3_org_equilibrium - C3_org); 
dC3_aq_dt  = (fPLSS/V3)*(cPLS - C3_aq)        - K_mass_3*(C3_org_equilibrium - C3_org);

end
